simulink model "TC_Conveyor"  (Simulink 8.1)
settings: Solver=ode45  StartTime=0.0  StopTime=9000.0  RelTol=1e-3
undefined symbols (not defined in the file or in its folder): rc_global, rc_input, rc_output, rc_switch_2TO1, rc_swith_1TO1, rc_sysAct, rc_sysAct1, rc_sysAct2, rc_sysAct3, rc_sysAct4, rc_sysAct5
settings Model: Creator=obo  LastModifiedBy=zhangpn
settings DataIOCC: SignalLoggingSaveFormat=Dataset
settings OptimizationCC: ExpressionDepthLimit=128
settings DebuggingCC: UnderspecifiedInitializationDetection=Simplified  FcnCallInpInsideContextMsg=EnableAllAsError  StateNameClashWarn=none
settings GRTTargetCC: CodeReplacementLibrary=None  CombineOutputUpdateFcns=on  CPPClassGenCompliant=on  GRTInterface=off

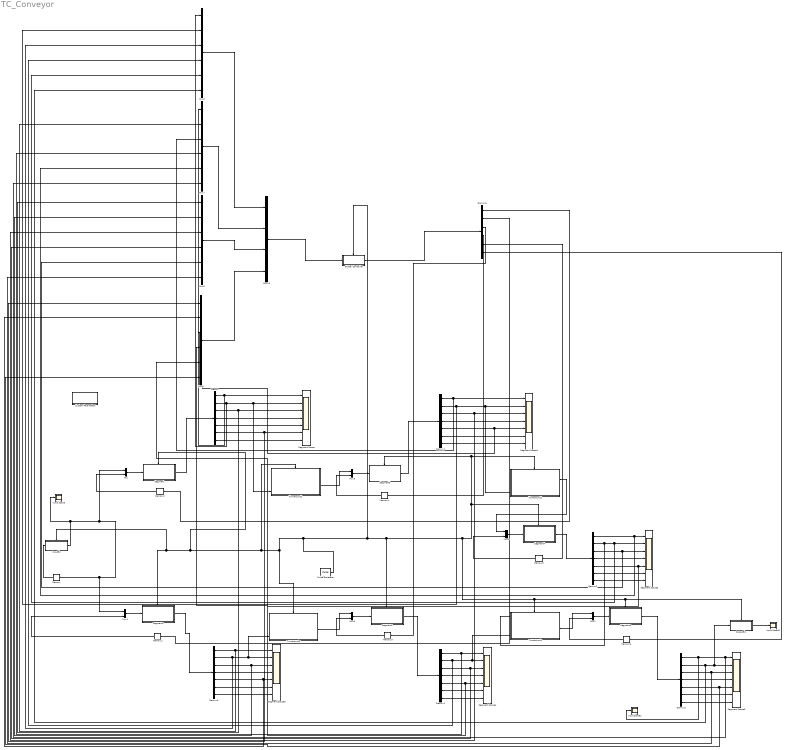
== system TC_Conveyor ==
  Demux{,1..5} (6 alike) : Demux  Outputs=7
  Demux6 : Demux  Outputs=6
  "Global Controller " : Subsystem
  Input Scope : Scope
      settings: YMin=100  YMax=650
  Input Scope1 : Scope
      settings: TimeRange=9000  YMin=0  YMax=140000  SaveName=ScopeData8
  Input Scope2 : Scope
      settings: TimeRange=9000  YMin=1.7e+06  YMax=3.7e+06  SaveName=ScopeData5
  InputBin : Subsystem
  Memory{,1..6} (7 alike) : Memory
  Mux{,1..5} (6 alike) : Mux  Inputs=2
  Mux10 : Mux
  Mux{6..9} (4 alike) : Mux  Inputs=6
  OutputBin : Subsystem
  Pulse Generator : DiscretePulseGenerator  PulseType=Time based  Period=1  PulseWidth=50  PhaseDelay=0.01
  Segment : Subsystem  TreatAsAtomicUnit=on
  Segment Scope{,1..5} (6 alike) : Scope  NumInputPorts=7
      Segment Scope settings: TimeRange=9000  YMin=150~150~950~475000~150~0.95~-1  YMax=400~400~1050~525000~400~1.05~1  MaxDataPoints=10000
      Segment Scope1 settings: TimeRange=9000  YMin=0~50~200~50000~50~0.25~-30  YMax=1750~450~425~350000~400~0.55~30  SaveName=ScopeData2  MaxDataPoints=10000
      Segment Scope2 settings: TimeRange=9000  YMin=100~100~200~2.77556e-17~100~0.2~-75  YMax=700~700~1000~0.5~700~1~75  SaveName=ScopeData3  MaxDataPoints=10000
      Segment Scope3 settings: TimeRange=9000  YMin=450~450~991.61~517521~450~0.495805~-40  YMax=800~800~1095.99~571997~800~0.547995~50  SaveName=ScopeData4  MaxDataPoints=10000
      Segment Scope4 settings: TimeRange=9000  YMin=0~0~2~5~5.55112e-17~0~0.2  YMax=35~150~8~25~1~700~1  SaveName=ScopeData6  MaxDataPoints=10000
      Segment Scope5 settings: TimeRange=9000  YMin=100~100~3966.44~8.28034e+06~100~0.495805~-30  YMax=450~450~4383.96~9.15196e+06~450~0.547995~30  SaveName=ScopeData7  MaxDataPoints=10000
  Segment1 : Subsystem  TreatAsAtomicUnit=on
  Segment2 : Subsystem  TreatAsAtomicUnit=on
  Segment3 : Subsystem  TreatAsAtomicUnit=on
  Segment4 : Subsystem  TreatAsAtomicUnit=on
  Segment5 : Subsystem  TreatAsAtomicUnit=on
  System Parameters : Subsystem  mask(Initialization Block){}
      mask help: Calls sc_init.m on it's initialization to declare and initialize all global variables.
      mask init:
      | rc_init
      mask Display: disp('Initialization')
  "Turnaround1 " : Subsystem
  Turnaround2 : Subsystem
  Turnaround3 : Subsystem
  "Turnaround4 " : Subsystem
  wires:
  Memory/1 -> InputBin/1(In1)
  Segment/1(sys_state) -> Demux/1
  Mux/1 -> Segment/1(Control_input)
  Segment1/1(sys_state) -> Demux3/1
  Mux1/1 -> Segment1/1(Control_input)
  "Turnaround4 "/3(EastOut) -> Mux2/1
  Segment5/1(sys_state) -> Demux5/1
  Mux2/1 -> Segment5/1(Control_input)
  OutputBin/1(Out1) -> Input Scope2/1
  Segment3/1(sys_state) -> Demux1/1
  Mux3/1 -> Segment3/1(Control_input)
  "Turnaround1 "/3(EastOut) -> Mux3/1
  Segment4/1(sys_state) -> Demux2/1
  Mux4/1 -> Segment4/1(Control_input)
  Turnaround2/2(SouthOut) -> Mux4/1
  Segment2/1(sys_state) -> Demux4/1
  Mux5/1 -> Segment2/1(Control_input)
  Turnaround3/3(EastOut) -> Mux5/1
  Pulse Generator/1 -> Turnaround3/Trigger, Segment1/Trigger, InputBin/Trigger, Segment/Trigger, "Turnaround1 "/Trigger, "Global Controller "/Trigger, Segment3/Trigger, Turnaround2/Trigger, Segment4/Trigger, "Turnaround4 "/Trigger, OutputBin/Trigger, Segment5/Trigger, Segment2/Trigger
  Demux/7 -> Segment Scope/7
  Demux/1 -> Mux7/1, Segment Scope/1
  Demux/3 -> Mux8/1, Segment Scope/3
  Demux/4 -> Segment Scope/4
  Demux/5 -> Segment Scope/5
  Demux/6 -> Mux9/1, Segment Scope/6
  Demux1/3 -> Mux8/3, Segment Scope1/3
  Demux1/1 -> Mux7/3, Segment Scope1/1
  Demux1/4 -> Segment Scope1/4
  Demux1/5 -> Mux9/3, Segment Scope1/5
  Demux1/6 -> Segment Scope1/6
  Demux1/7 -> Segment Scope1/7
  Demux3/1 -> Mux7/2, Segment Scope5/1
  Demux3/3 -> Mux8/2, Segment Scope5/3
  Demux3/4 -> Segment Scope5/4
  Demux3/5 -> Mux9/2, Segment Scope5/5
  Demux3/6 -> Segment Scope5/6
  Demux3/7 -> Segment Scope5/7
  Demux4/1 -> Mux7/4, Segment Scope4/1
  Demux4/3 -> Mux8/4, Segment Scope4/3
  Demux4/4 -> Segment Scope4/4
  Demux4/5 -> Mux9/5, Segment Scope4/5
  Demux4/6 -> Segment Scope4/6
  Demux4/7 -> Segment Scope4/7
  Demux2/1 -> Mux7/5, Segment Scope2/1
  Demux2/3 -> Mux8/5, Segment Scope2/3
  Demux2/4 -> Segment Scope2/4
  Demux2/5 -> Mux9/4, Segment Scope2/5
  Demux2/6 -> Segment Scope2/6
  Demux2/7 -> Segment Scope2/7
  Demux5/3 -> Mux8/6, Segment Scope3/3
  Demux5/4 -> Segment Scope3/4
  Demux5/5 -> Mux9/6, Segment Scope3/5
  Demux5/6 -> Segment Scope3/6
  Demux5/7 -> Segment Scope3/7
  Demux5/1 -> Input Scope1/1, Mux7/6, Segment Scope3/1
  InputBin/1(Out1) -> Mux/1, Mux1/1, Memory/1, Input Scope/1
  Demux1/2 -> Mux6/2, Turnaround2/4(WestIn), Segment Scope1/2
  Demux/2 -> Mux6/1, "Turnaround1 "/4(WestIn), Segment Scope/2
  Demux3/2 -> Mux6/3, Turnaround3/4(WestIn), Segment Scope5/2
  Demux4/2 -> Mux6/4, "Turnaround4 "/4(WestIn), Segment Scope4/2
  Demux2/2 -> "Turnaround4 "/1(NorthIn), Mux6/5, Segment Scope2/2
  Demux5/2 -> Mux6/6, OutputBin/1(In1), Segment Scope3/2
  "Global Controller "/1(Out1) -> Demux6/1
  Mux6/1 -> Mux10/1
  Mux7/1 -> Mux10/2
  Mux8/1 -> Mux10/3
  Mux9/1 -> Mux10/4
  Mux10/1 -> "Global Controller "/1(In1)
  Demux6/1 -> Memory2/1
  Memory2/1 -> Mux/2
  Demux6/2 -> Memory1/1
  Memory1/1 -> Mux1/2
  Demux6/3 -> Memory3/1
  Memory3/1 -> Mux5/2
  Demux6/4 -> Memory4/1
  Memory4/1 -> Mux3/2
  Demux6/5 -> Memory5/1
  Memory5/1 -> Mux4/2
  Demux6/6 -> Memory6/1
  Memory6/1 -> Mux2/2

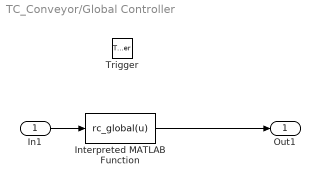
== system TC_Conveyor/Global Controller  ==
  In1 : Inport
  Trigger : TriggerPort  TriggerType=falling  PortDimensions=1
  Interpreted MATLAB Function : MATLABFcn  MATLABFcn=rc_global(u)  OutputDimensions=1*6
  Out1 : Outport  InitialOutput=[0]
  wires:
  In1/1 -> Interpreted MATLAB Function/1
  Interpreted MATLAB Function/1 -> Out1/1

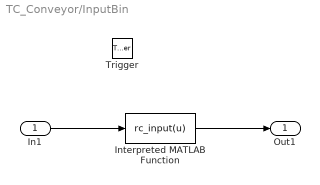
== system TC_Conveyor/InputBin ==
  In1 : Inport
  Trigger : TriggerPort  TriggerType=falling  PortDimensions=1
  Interpreted MATLAB Function : MATLABFcn  MATLABFcn=rc_input(u)  OutputDimensions=1
  Out1 : Outport  InitialOutput=[0]
  wires:
  In1/1 -> Interpreted MATLAB Function/1
  Interpreted MATLAB Function/1 -> Out1/1

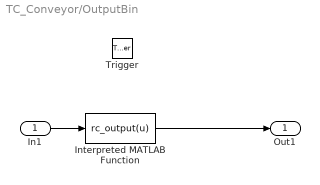
== system TC_Conveyor/OutputBin ==
  In1 : Inport
  Trigger : TriggerPort  TriggerType=falling  PortDimensions=1
  Interpreted MATLAB Function : MATLABFcn  MATLABFcn=rc_output(u)
  Out1 : Outport  InitialOutput=[0]
  wires:
  In1/1 -> Interpreted MATLAB Function/1
  Interpreted MATLAB Function/1 -> Out1/1

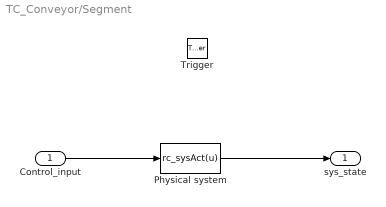
== system TC_Conveyor/Segment ==
  Control_input : Inport
  Trigger : TriggerPort  PortDimensions=1
  Physical system : MATLABFcn  MATLABFcn=rc_sysAct(u)  OutputDimensions=1*7  Output1D=off
  sys_state : Outport  InitialOutput=0
  wires:
  Control_input/1 -> Physical system/1
  Physical system/1 -> sys_state/1

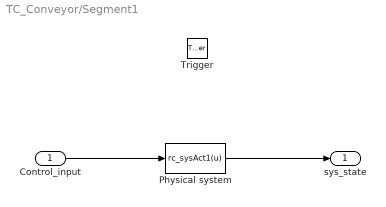
== system TC_Conveyor/Segment1 ==
  Control_input : Inport
  Trigger : TriggerPort  PortDimensions=1
  Physical system : MATLABFcn  MATLABFcn=rc_sysAct1(u)  OutputDimensions=1*7  Output1D=off
  sys_state : Outport  InitialOutput=0
  wires:
  Control_input/1 -> Physical system/1
  Physical system/1 -> sys_state/1

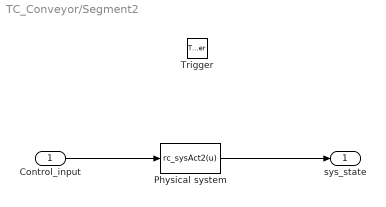
== system TC_Conveyor/Segment2 ==
  Control_input : Inport
  Trigger : TriggerPort  PortDimensions=1
  Physical system : MATLABFcn  MATLABFcn=rc_sysAct2(u)  OutputDimensions=1*7  Output1D=off
  sys_state : Outport  InitialOutput=0
  wires:
  Control_input/1 -> Physical system/1
  Physical system/1 -> sys_state/1

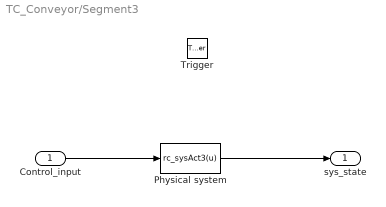
== system TC_Conveyor/Segment3 ==
  Control_input : Inport
  Trigger : TriggerPort  PortDimensions=1
  Physical system : MATLABFcn  MATLABFcn=rc_sysAct3(u)  OutputDimensions=1*7  Output1D=off
  sys_state : Outport  InitialOutput=0
  wires:
  Control_input/1 -> Physical system/1
  Physical system/1 -> sys_state/1

== system TC_Conveyor/Segment4 ==
  Control_input : Inport
  Trigger : TriggerPort  PortDimensions=1
  Physical system : MATLABFcn  MATLABFcn=rc_sysAct4(u)  OutputDimensions=1*7  Output1D=off
  sys_state : Outport  InitialOutput=0
  wires:
  Control_input/1 -> Physical system/1
  Physical system/1 -> sys_state/1

== system TC_Conveyor/Segment5 ==
  Control_input : Inport
  Trigger : TriggerPort  PortDimensions=1
  Physical system : MATLABFcn  MATLABFcn=rc_sysAct5(u)  OutputDimensions=1*7  Output1D=off
  sys_state : Outport  InitialOutput=0
  wires:
  Control_input/1 -> Physical system/1
  Physical system/1 -> sys_state/1

== system TC_Conveyor/System Parameters ==

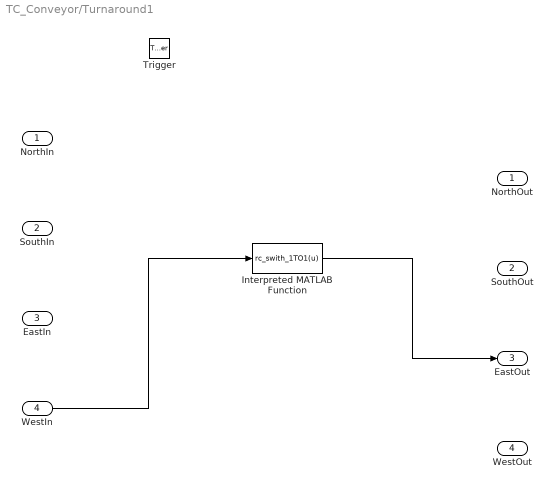
== system TC_Conveyor/Turnaround1  ==
  NorthIn : Inport
  SouthIn : Inport  Port=2
  EastIn : Inport  Port=3
  WestIn : Inport  Port=4
  Trigger : TriggerPort  TriggerType=falling  PortDimensions=1
  Interpreted MATLAB Function : MATLABFcn  MATLABFcn=rc_swith_1TO1(u)
  NorthOut : Outport  InitialOutput=[0]
  SouthOut : Outport  Port=2  InitialOutput=[0]
  EastOut : Outport  Port=3  InitialOutput=[0]
  WestOut : Outport  Port=4  InitialOutput=[0]
  wires:
  WestIn/1 -> Interpreted MATLAB Function/1
  Interpreted MATLAB Function/1 -> EastOut/1

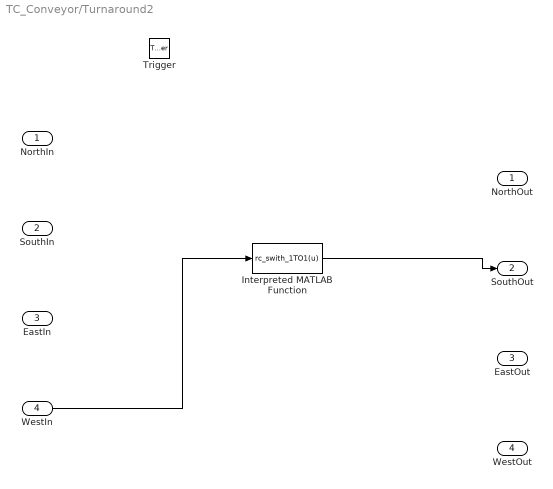
== system TC_Conveyor/Turnaround2 ==
  NorthIn : Inport
  SouthIn : Inport  Port=2
  EastIn : Inport  Port=3
  WestIn : Inport  Port=4
  Trigger : TriggerPort  TriggerType=falling  PortDimensions=1
  Interpreted MATLAB Function : MATLABFcn  MATLABFcn=rc_swith_1TO1(u)
  NorthOut : Outport  InitialOutput=[0]
  SouthOut : Outport  Port=2  InitialOutput=[0]
  EastOut : Outport  Port=3  InitialOutput=[0]
  WestOut : Outport  Port=4  InitialOutput=[0]
  wires:
  WestIn/1 -> Interpreted MATLAB Function/1
  Interpreted MATLAB Function/1 -> SouthOut/1

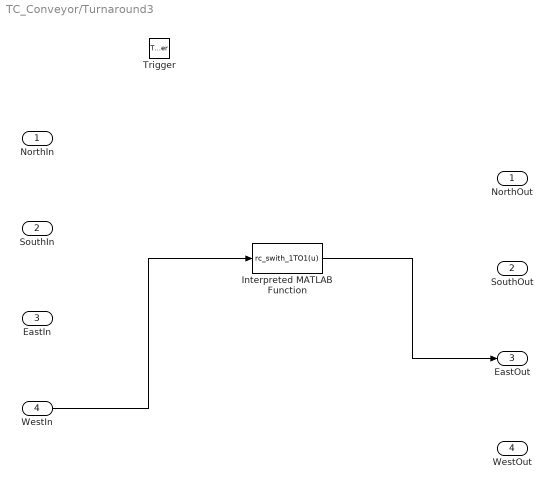
== system TC_Conveyor/Turnaround3 ==
  NorthIn : Inport
  SouthIn : Inport  Port=2
  EastIn : Inport  Port=3
  WestIn : Inport  Port=4
  Trigger : TriggerPort  TriggerType=falling  PortDimensions=1
  Interpreted MATLAB Function : MATLABFcn  MATLABFcn=rc_swith_1TO1(u)
  NorthOut : Outport  InitialOutput=[0]
  SouthOut : Outport  Port=2  InitialOutput=[0]
  EastOut : Outport  Port=3  InitialOutput=[0]
  WestOut : Outport  Port=4  InitialOutput=[0]
  wires:
  WestIn/1 -> Interpreted MATLAB Function/1
  Interpreted MATLAB Function/1 -> EastOut/1

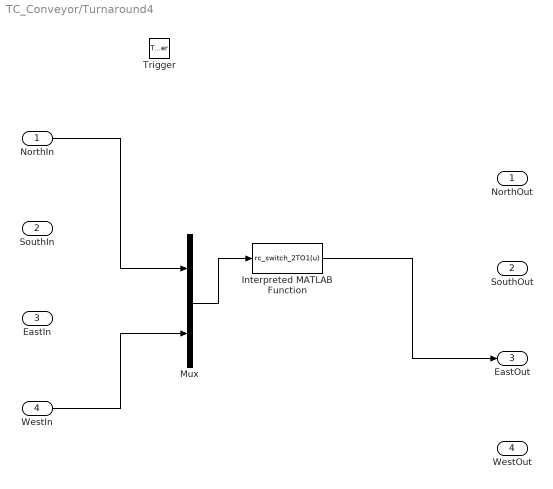
== system TC_Conveyor/Turnaround4  ==
  NorthIn : Inport
  SouthIn : Inport  Port=2
  EastIn : Inport  Port=3
  WestIn : Inport  Port=4
  Trigger : TriggerPort  TriggerType=falling  PortDimensions=1
  Interpreted MATLAB Function : MATLABFcn  MATLABFcn=rc_switch_2TO1(u)
  Mux : Mux  Inputs=2
  NorthOut : Outport  InitialOutput=[0]
  SouthOut : Outport  Port=2  InitialOutput=[0]
  EastOut : Outport  Port=3  InitialOutput=[0]
  WestOut : Outport  Port=4  InitialOutput=[0]
  wires:
  WestIn/1 -> Mux/2
  NorthIn/1 -> Mux/1
  Mux/1 -> Interpreted MATLAB Function/1
  Interpreted MATLAB Function/1 -> EastOut/1
